simulink model "inverter"  (R2021a)
settings: Solver=VariableStepAuto  StartTime=0.0  StopTime=10.0  RelTol=1e-3
settings Model: Creator=zager  LastModifiedBy=zager

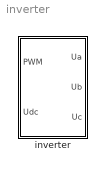
== system inverter ==
  inverter : Subsystem

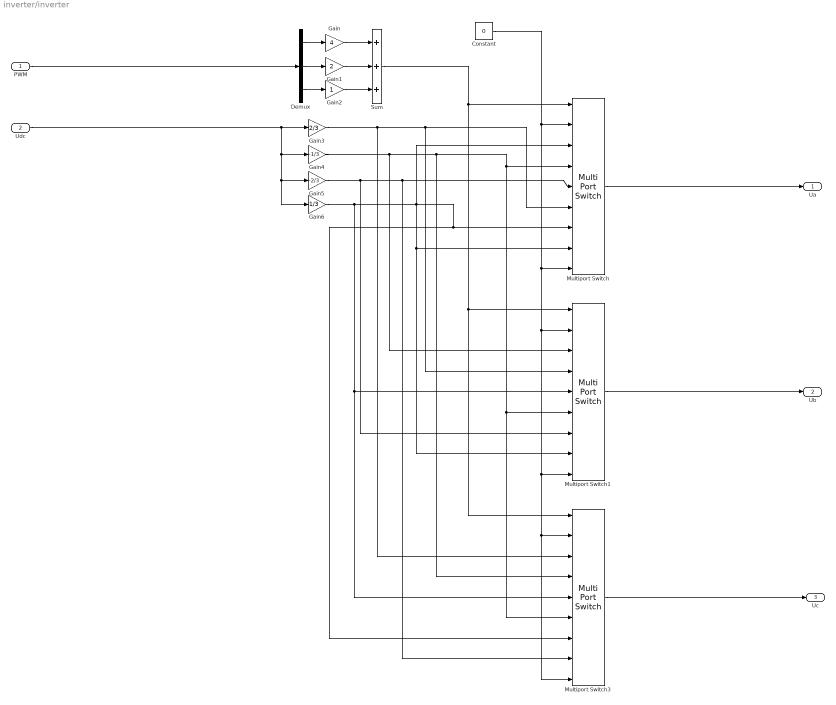
== system inverter/inverter ==
  PWM : Inport
  Udc : Inport  Port=2
  Constant : Constant  Value=0
  Demux : Demux  Outputs=3
  Gain : Gain  Gain=4
  Gain1 : Gain  Gain=2
  Gain2 : Gain
  Gain3 : Gain  Gain=2/3
  Gain4 : Gain  Gain=-1/3
  Gain5 : Gain  Gain=-2/3
  Gain6 : Gain  Gain=1/3
  Multiport Switch : MultiPortSwitch  DataPortOrder=Zero-based contiguous  Inputs=8  zeroidx=on
  Multiport Switch1 : MultiPortSwitch  DataPortOrder=Zero-based contiguous  Inputs=8  zeroidx=on
  Multiport Switch3 : MultiPortSwitch  DataPortOrder=Zero-based contiguous  Inputs=8  zeroidx=on
  Sum : Sum  Inputs=+++
  Ua : Outport
  Ub : Outport  Port=2
  Uc : Outport  Port=3
  wires:
  Gain6/1 -> Multiport Switch3/5, Multiport Switch1/5, Multiport Switch3/7, Multiport Switch/7, Multiport Switch1/8, Multiport Switch/8, Multiport Switch/3
  Gain5/1 -> Multiport Switch1/7, Multiport Switch/5, Multiport Switch3/8
  PWM/1 -> Demux/1
  Udc/1 -> Gain6/1, Gain5/1, Gain4/1, Gain3/1
  Demux/2 -> Gain1/1
  Gain/1 -> Sum/1
  Gain3/1 -> Multiport Switch3/3, Multiport Switch1/4, Multiport Switch/6
  Sum/1 -> Multiport Switch3/1, Multiport Switch1/1, Multiport Switch/1
  Gain4/1 -> Multiport Switch1/3, Multiport Switch3/4, Multiport Switch1/6, Multiport Switch3/6, Multiport Switch/4
  Gain2/1 -> Sum/3
  Constant/1 -> Multiport Switch3/9, Multiport Switch3/2, Multiport Switch1/9, Multiport Switch1/2, Multiport Switch/9, Multiport Switch/2
  Demux/1 -> Gain/1
  Gain1/1 -> Sum/2
  Multiport Switch/1 -> Ua/1
  Demux/3 -> Gain2/1
  Multiport Switch1/1 -> Ub/1
  Multiport Switch3/1 -> Uc/1
